simulink model "appollo_model"  (R2014a)
settings: Solver=ode45  StartTime=0.0  StopTime=10.0  RelTol=1e-3
values from neighbouring files (symbols this model uses):
  mu = 1/82.45    (= 0.0121285627653)    [appollo.m]
undefined symbols (not defined in the file or in its folder): mu1
libraries: simulink x1
settings Model: Creator=chaor  LastModifiedBy=chaor
settings DataIOCC: InspectSignalLogs=on

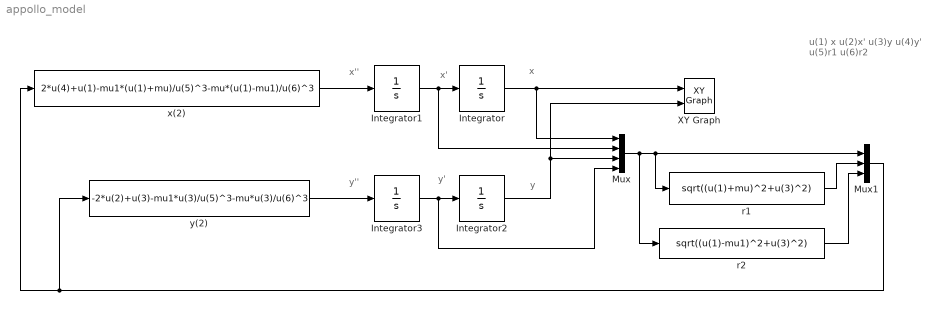
== system appollo_model ==
  note: u(1) x
      | u(2)x'
      | u(3)y
      | u(4)y'
      | u(5)r1
      | u(6)r2
  note: y''
  note: y'
  note: y
  note: x''
  note: x'
  note: x
  Integrator : Integrator  InitialCondition=1.2
  Integrator1 : Integrator
  Integrator2 : Integrator
  Integrator3 : Integrator  InitialCondition=-1.04935751
  Mux : Mux
  Mux1 : Mux  Inputs=3
  XY Graph : simulink/Sinks/XY Graph  xmin=-1.5  xmax=1.5  ymin=-0.8  ymax=0.8  st=-1
  "r1 " : Fcn  Expr=sqrt((u(1)+mu)^2+u(3)^2)
  "r2 " : Fcn  Expr=sqrt((u(1)-mu1)^2+u(3)^2)
  x(2) : Fcn  Expr=2*u(4)+u(1)-mu1*(u(1)+mu)/u(5)^3-mu*(u(1)-mu1)/u(6)^3
  y(2) : Fcn  Expr=-2*u(2)+u(3)-mu1*u(3)/u(5)^3-mu*u(3)/u(6)^3
  wires:
  Integrator/1 -> XY Graph/1, Mux/1
  Integrator1/1 -> Mux/2, Integrator/1
  Integrator3/1 -> Mux/4, Integrator2/1
  x(2)/1 -> Integrator1/1
  y(2)/1 -> Integrator3/1
  Integrator2/1 -> XY Graph/2, Mux/3
  Mux/1 -> "r2 "/1, "r1 "/1, Mux1/1
  "r1 "/1 -> Mux1/2
  "r2 "/1 -> Mux1/3
  Mux1/1 -> x(2)/1, y(2)/1
